simulink model "AutomatedParkingValet"  (R2022b)
settings: Solver=ode23tb  StartTime=0.0  StopTime=inf  FixedStep=1e-3  MaxStep=1e-2  MinStep=1e-3  RelTol=5e-3
PreLoadFcn:
  | costmap = helperSLCreateCostmap();
  | routeData= load('routePlanSL.mat');
  | routePlan= routeData.routePlan;
  | startPose = routePlan.StartPose(1, :);
  | centerToFront = 1.4;
  | centerToRear = 1.4;
  | helperSLCreateUtilityBus;
StopFcn:
  | clear helperSLVisualizePath
libraries: drivinglib x2, simulink x2, simulink_extras x2, autolibshared x1
CloseFcn:
  | clear plannerConfigBus ...
  | speedConfigBus ...
  | startPose ...
  | costmap ...
  | routeData ...
  | routePlan ...
  | centerToFront ...
  | centerToRear;
settings Model: Creator=The MathWorks, Inc.  LastModifiedBy=The MathWorks, Inc.
settings SolverCC: ZeroCrossAlgorithm=Adaptive  AlgebraicLoopSolver=TrustRegion  DecoupledContinuousIntegration=on  MinimalZcImpactIntegration=on
settings DataIOCC: SaveOutput=off  SignalLogging=off  DSMLogging=off  SaveTime=off  ReturnWorkspaceOutputs=off
settings DebuggingCC: UnconnectedInputMsg=warning  UnconnectedOutputMsg=warning  UnconnectedLineMsg=warning  PregeneratedLibrarySubsystemCodeDiagnostic=none  SFMachineParentedDataDiag=warning  ArithmeticOperatorsInVariantConditions=warning
settings ModelReferenceCC: EnableRefExpFcnMdlSchedulingChecks=on
settings SFSimCC: SimUseLocalCustomCode=off
settings RTWCC: RTWUseLocalCustomCode=off

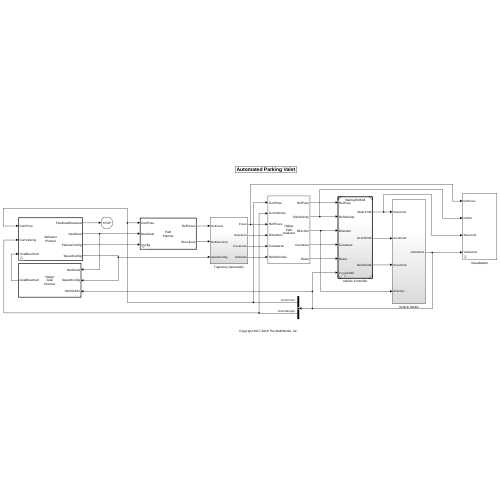
[thumbnail: Simulink's stored preview of the top-level diagram]
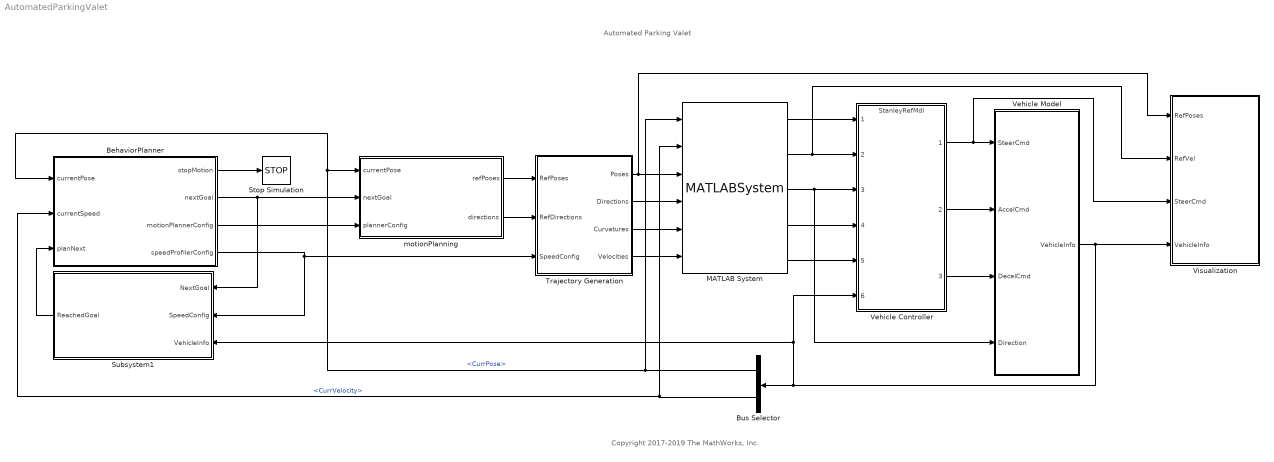
== system AutomatedParkingValet ==
  note: Copyright 2017-2019 The MathWorks, Inc.
  note: Automated Parking Valet
  BehaviorPlanner : MATLAB Function  TreatAsAtomicUnit=on  mask{Costmap=costmap, RoutePlan=routePlan, StartSpeed=0}
      mask prompts: Costmap "Vehicle costmap:"; RoutePlan "Route plan:"; StartSpeed "Initial vehicle speed  [m/s]:"
      mask init:
      | validateattributes(Costmap, {'vehicleCostmap'}, {'scalar'});
      | validateattributes(RoutePlan, {'table'}, {'ncols', 3});
      | validateattributes(StartSpeed, {'double'}, {'scalar','nonnegative'})
      | 
      | routePlanStruct   = table2struct(RoutePlan);
      | startPose         = routePlanStruct(1).StartPose;
      | 
      | varagout          = helperSLCreateUtilityStruct(Costmap);
      | vehicleDimsStruct = varagout{1};
      | costmapStruct     = varagout{2};
  Bus Selector : BusSelector  OutputSignals=CurrPose,CurrVelocity
  MATLAB System : MATLABSystem  System=HelperPathAnalyzer  Wheelbase=2.8  HasResetOutput=on  SimulateUsing=Interpreted execution
      mask Type: HelperPathAnalyzer
      mask Display:
      | disp(['Helper' char(10) 'Path' char(10) 'Analyzer']);
      | port_label('input',1,'CurrPose');
      | port_label('input',2,'CurrVelocity');
      | port_label('input',3,'RefPoses');
      | port_label('input',4,'Directions');
      | port_label('input',5,'Curvatures');
      | port_label('input',6,'RefVelocities');
      | port_label('output',1,'RefPose');
      | port_label('output',2,'RefVelocity');
      | port_label('output',3,'Direction');
      | port_label('output',4,'Curvature');
      | port_label('output',5,'Reset');
  Stop Simulation : Stop
  Subsystem1 : Subsystem  TreatAsAtomicUnit=on  SystemSampleTime=0.1
      settings: MinAlgLoopOccurrences=on
      mask Display:
      | disp(['Helper' char(10) 'Goal' char(10) 'Checker']);
      | port_label('input',1,'NextGoal');
      | port_label('input',2,'SpeedConfig');
      | port_label('input',3,'VehicleInfo');
      | port_label('output',1,'GoalReached');
  Trajectory Generation : Subsystem
  Vehicle Controller : ModelReference  ModelNameDialog=StanleyRefMdl  SimulationMode=Normal  ModelReferenceVersion=1.948
  Vehicle Model : Subsystem
  Visualization : Subsystem  mask{Costmap=costmap}
      mask prompts: Costmap "Vehicle costmap:"
      mask init:
      | validateattributes(Costmap, {'vehicleCostmap'}, {'scalar'});
      | 
      | varagout          = helperSLCreateUtilityStruct(Costmap);
      | vehicleDimsStruct = varagout{1};
      | costmapStruct     = varagout{2};
      mask DialogControl DescTextVar Prompt: Visualize simulation results.
  motionPlanning : MATLAB Function  TreatAsAtomicUnit=on  mask{Costmap=costmap}
      mask prompts: Costmap "Vehicle costmap:"
      mask init:
      | validateattributes(Costmap, {'vehicleCostmap'}, {'scalar'});
      | 
      | varagout          = helperSLCreateUtilityStruct(Costmap);
      | vehicleDimsStruct = varagout{1};
      | costmapStruct     = varagout{2};
  wires:
  BehaviorPlanner/2(nextGoal) -> Subsystem1/1(NextGoal), motionPlanning/2(nextGoal)
  BehaviorPlanner/3(motionPlannerConfig) -> motionPlanning/3(plannerConfig)
  BehaviorPlanner/1(stopMotion) -> Stop Simulation/1
  BehaviorPlanner/4(speedProfilerConfig) -> Subsystem1/2(SpeedConfig), Trajectory Generation/3(SpeedConfig)
  Subsystem1/1(ReachedGoal) -> BehaviorPlanner/3(planNext)
  MATLAB System/3 -> Vehicle Controller/3, Vehicle Model/4(Direction)
  MATLAB System/2 -> Vehicle Controller/2, Visualization/2(RefVel)
  MATLAB System/1 -> Vehicle Controller/1
  MATLAB System/4 -> Vehicle Controller/4
  Vehicle Model/1(VehicleInfo) -> Vehicle Controller/6, Subsystem1/3(VehicleInfo), Bus Selector/1, Visualization/4(VehicleInfo)
  Bus Selector/1 -> BehaviorPlanner/1(currentPose), motionPlanning/1(currentPose), MATLAB System/1  "<CurrPose>"
  Bus Selector/2 -> MATLAB System/2, BehaviorPlanner/2(currentSpeed)  "<CurrVelocity>"
  MATLAB System/5 -> Vehicle Controller/5
  Vehicle Controller/3 -> Vehicle Model/3(DecelCmd)
  Vehicle Controller/1 -> Vehicle Model/1(SteerCmd), Visualization/3(SteerCmd)
  Vehicle Controller/2 -> Vehicle Model/2(AccelCmd)
  Trajectory Generation/1(Poses) -> Visualization/1(RefPoses), MATLAB System/3
  motionPlanning/1(refPoses) -> Trajectory Generation/1(RefPoses)
  motionPlanning/2(directions) -> Trajectory Generation/2(RefDirections)
  Trajectory Generation/2(Directions) -> MATLAB System/4
  Trajectory Generation/3(Curvatures) -> MATLAB System/5
  Trajectory Generation/4(Velocities) -> MATLAB System/6

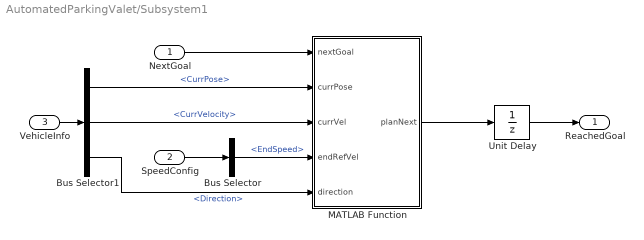
== system AutomatedParkingValet/Subsystem1 ==
  NextGoal : Inport
  SpeedConfig : Inport  Port=2
  VehicleInfo : Inport  Port=3
  Bus Selector : BusSelector  OutputSignals=EndSpeed
  Bus Selector1 : BusSelector  OutputSignals=CurrPose,CurrVelocity,Direction
  MATLAB Function : MATLAB Function  TreatAsAtomicUnit=on
  Unit Delay : UnitDelay  SampleTime=-1  HasFrameUpgradeWarning=on
  ReachedGoal : Outport  VectorParamsAs1DForOutWhenUnconnected=off
  wires:
  Bus Selector1/1 -> MATLAB Function/2(currPose)  "<CurrPose>"
  VehicleInfo/1 -> Bus Selector1/1
  Bus Selector1/3 -> MATLAB Function/5(direction)  "<Direction>"
  Bus Selector/1 -> MATLAB Function/4(endRefVel)  "<EndSpeed>"
  Unit Delay/1 -> ReachedGoal/1
  SpeedConfig/1 -> Bus Selector/1
  MATLAB Function/1(planNext) -> Unit Delay/1
  Bus Selector1/2 -> MATLAB Function/3(currVel)  "<CurrVelocity>"
  NextGoal/1 -> MATLAB Function/1(nextGoal)

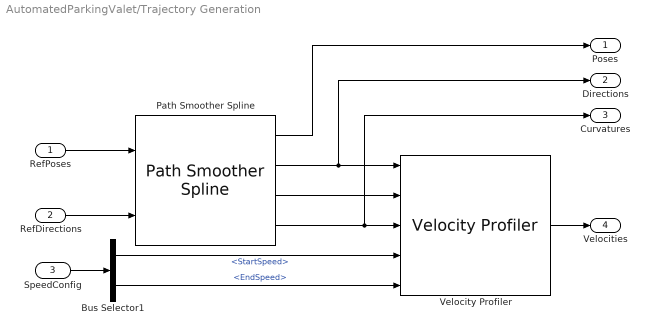
== system AutomatedParkingValet/Trajectory Generation ==
  RefPoses : Inport
  RefDirections : Inport  Port=2
  SpeedConfig : Inport  Port=3
  Bus Selector1 : BusSelector  OutputSignals=StartSpeed,EndSpeed
  Path Smoother Spline : drivinglib/Path Smoother Spline  NumSmoothPoses=500  MinSeparation=1e-3  SampleTime=-1  ShowOptionalOutports=on  SimulateUsing=Interpreted execution
  Velocity Profiler : drivinglib/Velocity Profiler  MaxLongitudinalAccel=2  MaxLongitudinalDecel=4  MaxSpeed=10  MaxLongitudinalJerk=1  MaxLateralAccel=2  ShowOptionalOutport=off  SampleTime=-1  SimulateUsing=Interpreted execution
  Poses : Outport  VectorParamsAs1DForOutWhenUnconnected=off
  Directions : Outport  Port=2  VectorParamsAs1DForOutWhenUnconnected=off
  Curvatures : Outport  Port=3  VectorParamsAs1DForOutWhenUnconnected=off
  Velocities : Outport  Port=4  VectorParamsAs1DForOutWhenUnconnected=off
  wires:
  Velocity Profiler/1 -> Velocities/1
  Path Smoother Spline/2 -> Directions/1, Velocity Profiler/1
  Path Smoother Spline/4 -> Curvatures/1, Velocity Profiler/3
  Bus Selector1/2 -> Velocity Profiler/5  "<EndSpeed>"
  RefPoses/1 -> Path Smoother Spline/1
  SpeedConfig/1 -> Bus Selector1/1
  Bus Selector1/1 -> Velocity Profiler/4  "<StartSpeed>"
  Path Smoother Spline/3 -> Velocity Profiler/2
  RefDirections/1 -> Path Smoother Spline/2
  Path Smoother Spline/1 -> Poses/1

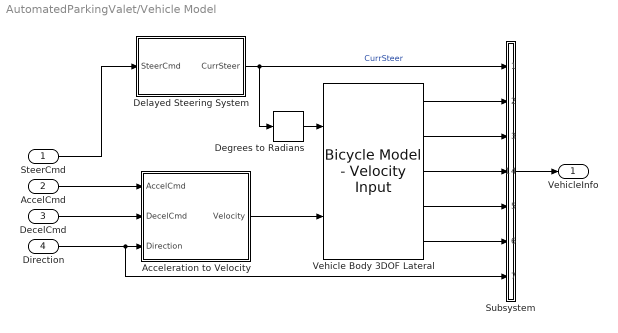
== system AutomatedParkingValet/Vehicle Model ==
  SteerCmd : Inport
  AccelCmd : Inport  Port=2
  DecelCmd : Inport  Port=3
  Direction : Inport  Port=4
  Acceleration to Velocity : Subsystem  TreatAsAtomicUnit=on
  Degrees to Radians : simulink_extras/Transformations/Degrees to Radians
  Delayed Steering System : Subsystem
  Subsystem : Subsystem
  Vehicle Body 3DOF Lateral : autolibshared/Bicycle Model - Velocity Input  trackMode=Single (bicycle)  inputMode=External longitudinal forces  frontSteerMode=on  rearSteerMode=off  windMode=off  muMode=off  extFMode=off  extMMode=off  aMode=3  NF=2  NR=2  m=1575  a=1.2  b=1.6  h=0.35  X_o=startPose(1)+cosd(startPose(3))*1.6  xdot_o=0  CalphaMode=off  sigmaMode=on  w=[1.4,1.4]  Cy_f=19e3  Cy_r=20e3  sigma_f=.1  sigma_r=.1  alpha_f_brk=[-.1 .1]  Cy_f_data=[-9e3 9e3]  alpha_r_brk=[-.1 .1]  Cy_r_data=[-9e3 9e3]  Y_o=startPose(2) +sind(startPose(3))*1.6  ydot_o=0  Izz=4000  psi_o=deg2rad(startPose(3))  r_o=0  Af=2  Cd=.3  Cl=.1  Cpm=.1  beta_w=[0:0.01:0.3]  Cs=[0:0.03:0.9]  Cym=[0:0.01:0.3]  Pabs=101325  Tair=273  g=9.81  mu=1  xdot_tol=0.01  Fznom=5000  Fxtire_sat=1e6  Fytire_sat=1e6  longOff=0  latOff=0  vertOff=0
  VehicleInfo : Outport  VectorParamsAs1DForOutWhenUnconnected=off
  wires:
  Acceleration to Velocity/1(Velocity) -> Vehicle Body 3DOF Lateral/2
  Direction/1 -> Subsystem/7(<Direction>), Acceleration to Velocity/3(Direction)
  Degrees to Radians/1 -> Vehicle Body 3DOF Lateral/1
  Delayed Steering System/1(CurrSteer) -> Degrees to Radians/1, Subsystem/1(CurrSteer)  "CurrSteer"
  DecelCmd/1 -> Acceleration to Velocity/2(DecelCmd)
  AccelCmd/1 -> Acceleration to Velocity/1(AccelCmd)
  SteerCmd/1 -> Delayed Steering System/1(SteerCmd)
  Subsystem/1(VehicleInfo) -> VehicleInfo/1
  Vehicle Body 3DOF Lateral/1 -> Subsystem/2(Info)
  Vehicle Body 3DOF Lateral/2 -> Subsystem/3(In3)
  Vehicle Body 3DOF Lateral/3 -> Subsystem/4(In4)
  Vehicle Body 3DOF Lateral/4 -> Subsystem/5(In5)
  Vehicle Body 3DOF Lateral/5 -> Subsystem/6(In6)

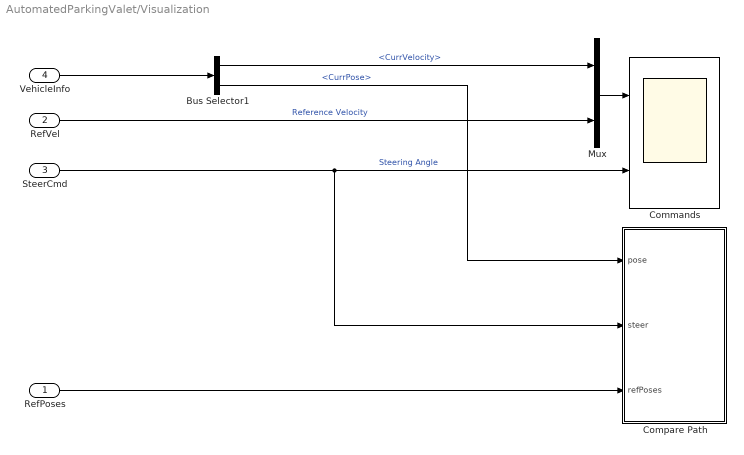
== system AutomatedParkingValet/Visualization ==
  RefPoses : Inport
  RefVel : Inport  Port=2
  SteerCmd : Inport  Port=3
  VehicleInfo : Inport  Port=4
  Bus Selector1 : BusSelector  OutputSignals=CurrVelocity,CurrPose
  Commands : Scope  NumInputPorts=2
  Compare Path : MATLAB Function  TreatAsAtomicUnit=on
  Mux : Mux  Inputs=2
  wires:
  RefPoses/1 -> Compare Path/3(refPoses)
  Bus Selector1/1 -> Mux/1  "<CurrVelocity>"
  Bus Selector1/2 -> Compare Path/1(pose)  "<CurrPose>"
  RefVel/1 -> Mux/2  "Reference Velocity"
  Mux/1 -> Commands/1
  SteerCmd/1 -> Compare Path/2(steer), Commands/2  "Steering Angle"
  VehicleInfo/1 -> Bus Selector1/1

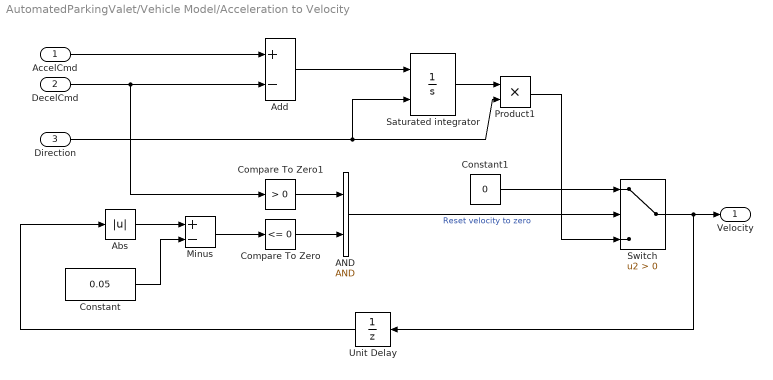
== system AutomatedParkingValet/Vehicle Model/Acceleration to Velocity ==
  AccelCmd : Inport  PortDimensions=[1 1]
  DecelCmd : Inport  Port=2  PortDimensions=[1 1]
  Direction : Inport  Port=3
  AND : Logic  IconShape=distinctive  AllPortsSameDT=off  OutDataTypeStr=boolean
  Abs : Abs  SaturateOnIntegerOverflow=off
  Add : Sum  Inputs=+-
  Compare To Zero : simulink/Logic and Bit Operations/Compare To Zero  relop=<=  OutDataTypeStr=boolean
  Compare To Zero1 : simulink/Logic and Bit Operations/Compare To Zero  relop=>  OutDataTypeStr=boolean
  Constant : Constant  Value=0.05
  Constant1 : Constant  Value=0
  Minus : Sum  Inputs=+-
  Product1 : Product
  Saturated integrator : Integrator  ExternalReset=either  LimitOutput=on  LowerSaturationLimit=0  AbsoluteTolerance=1e-3  ZeroCross=off
  Switch : Switch  Criteria=u2 > Threshold  SaturateOnIntegerOverflow=off  InputSameDT=off
  Unit Delay : UnitDelay  SampleTime=-1  HasFrameUpgradeWarning=on
  Velocity : Outport  VectorParamsAs1DForOutWhenUnconnected=off
  wires:
  Direction/1 -> Product1/2, Saturated integrator/2
  AccelCmd/1 -> Add/1
  Add/1 -> Saturated integrator/1
  DecelCmd/1 -> Compare To Zero1/1, Add/2
  Unit Delay/1 -> Abs/1
  Abs/1 -> Minus/1
  Constant/1 -> Minus/2
  Minus/1 -> Compare To Zero/1
  Compare To Zero/1 -> AND/2
  Compare To Zero1/1 -> AND/1
  AND/1 -> Switch/2  "Reset velocity to zero"
  Switch/1 -> Unit Delay/1, Velocity/1
  Constant1/1 -> Switch/1
  Saturated integrator/1 -> Product1/1
  Product1/1 -> Switch/3

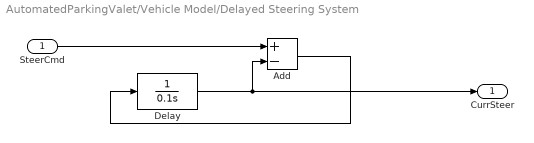
== system AutomatedParkingValet/Vehicle Model/Delayed Steering System ==
  SteerCmd : Inport
  Add : Sum  Inputs=+-
  Delay : TransferFcn  Denominator=[0.1 0]
  CurrSteer : Outport  VectorParamsAs1DForOutWhenUnconnected=off
  wires:
  Add/1 -> Delay/1
  SteerCmd/1 -> Add/1
  Delay/1 -> CurrSteer/1, Add/2

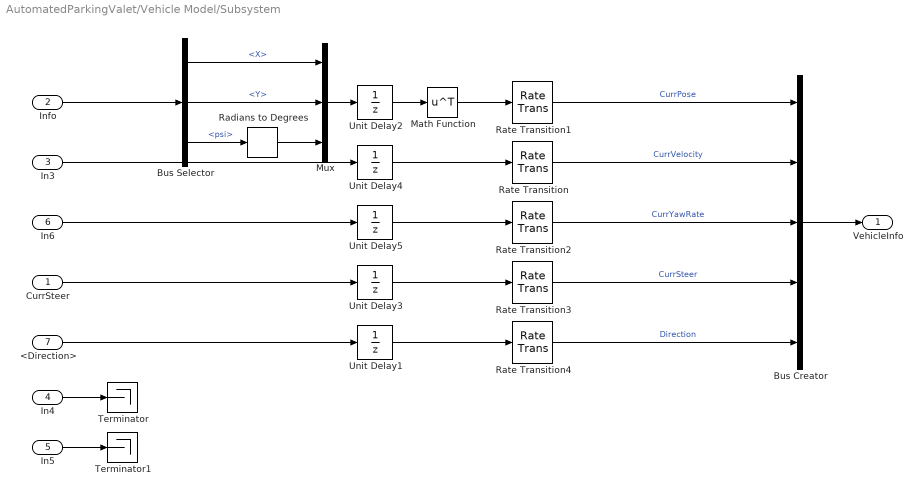
== system AutomatedParkingValet/Vehicle Model/Subsystem ==
  CurrSteer : Inport
  Info : Inport  Port=2
  In3 : Inport  Port=3
  In4 : Inport  Port=4
  In5 : Inport  Port=5
  In6 : Inport  Port=6
  <Direction> : Inport  Port=7
  Bus Creator : BusCreator  Inputs=5  OutDataTypeStr=Bus: vehicleInfoBus  NonVirtualBus=on
  Bus Selector : BusSelector  OutputSignals=InertFrm.RearAxl.Disp.X,InertFrm.RearAxl.Disp.Y,InertFrm.Cg.Ang.psi
  Math Function : Math  Operator=transpose  SignedPower=on
  Mux : Mux  Inputs=3
  Radians to Degrees : simulink_extras/Transformations/Radians to Degrees
  Rate Transition : RateTransition  OutPortSampleTime=0.05
  Rate Transition1 : RateTransition  InitialCondition=startPose  OutPortSampleTime=0.05
  Rate Transition2 : RateTransition  OutPortSampleTime=0.05
  Rate Transition3 : RateTransition  OutPortSampleTime=0.05
  Rate Transition4 : RateTransition  InitialCondition=1  OutPortSampleTime=0.05
  Terminator : Terminator
  Terminator1 : Terminator
  Unit Delay1 : UnitDelay  InitialCondition=1  SampleTime=-1  HasFrameUpgradeWarning=on
  Unit Delay2 : UnitDelay  InitialCondition=startPose  SampleTime=-1  HasFrameUpgradeWarning=on
  Unit Delay3 : UnitDelay  SampleTime=-1  HasFrameUpgradeWarning=on
  Unit Delay4 : UnitDelay  SampleTime=-1  HasFrameUpgradeWarning=on
  Unit Delay5 : UnitDelay  SampleTime=-1  HasFrameUpgradeWarning=on
  VehicleInfo : Outport  VectorParamsAs1DForOutWhenUnconnected=off
  wires:
  Unit Delay1/1 -> Rate Transition4/1
  CurrSteer/1 -> Unit Delay3/1
  Unit Delay5/1 -> Rate Transition2/1
  <Direction>/1 -> Unit Delay1/1
  Unit Delay4/1 -> Rate Transition/1
  Math Function/1 -> Rate Transition1/1
  Rate Transition/1 -> Bus Creator/2  "CurrVelocity"
  Unit Delay3/1 -> Rate Transition3/1
  Rate Transition3/1 -> Bus Creator/4  "CurrSteer"
  Rate Transition1/1 -> Bus Creator/1  "CurrPose"
  Rate Transition2/1 -> Bus Creator/3  "CurrYawRate"
  Rate Transition4/1 -> Bus Creator/5  "Direction"
  In5/1 -> Terminator1/1
  Unit Delay2/1 -> Math Function/1
  Info/1 -> Bus Selector/1
  Radians to Degrees/1 -> Mux/3
  Bus Selector/2 -> Mux/2  "<Y>"
  Bus Selector/1 -> Mux/1  "<X>"
  Mux/1 -> Unit Delay2/1
  In3/1 -> Unit Delay4/1
  In4/1 -> Terminator/1
  In6/1 -> Unit Delay5/1
  Bus Selector/3 -> Radians to Degrees/1  "<psi>"
  Bus Creator/1 -> VehicleInfo/1

== matlab function AutomatedParkingValet/motionPlanning ==
  settings: updateMethod=DISCRETE  sampleTime=0.1
  data: refPoses output size=[100 3]; currentPose input size=[1 3]; nextGoal input size=[1 3]; plannerConfig input Bus: plannerConfigBus; costmapStruct parameter; vehicleDimsStruct parameter; directions output size=[100 1]
function [refPoses, directions] = motionPlanning(currentPose, nextGoal, ...
    plannerConfig, costmapStruct, vehicleDimsStruct)

%motionPlanning plan a feasible path using pathPlannerRRT.

%#codegen

persistent nextGoalPose posesInternal directionsInternal

% Initialize persistent variables
if isempty(nextGoalPose)
    nextGoalPose = [0 0 0];
end

if isempty(posesInternal)
    posesInternal = [0 0 0];
end

if isempty(directionsInternal)
    directionsInternal = 1;
end

% Create vehicleDimensions object
vehicleDims = vehicleDimensions( ...
    vehicleDimsStruct.Length, ...
    vehicleDimsStruct.Width, ...
    vehicleDimsStruct.Height, ...
    'Wheelbase',          vehicleDimsStruct.Wheelbase, ...
    'RearOverhang',       vehicleDimsStruct.RearOverhang, ...
    'WorldUnits',         char(vehicleDimsStruct.WorldUnits));

ccConfig = inflationCollisionChecker(vehicleDims, 4);

% Initialize vehicleCostmap object
costmap = vehicleCostmap(costmapStruct.Costs, ...
    'FreeThreshold',      costmapStruct.FreeThreshold, ...
    'OccupiedThreshold',  costmapStruct.OccupiedThreshold, ...
    'MapLocation',        costmapStruct.MapExtent([1, 3]), ...
    'CellSize',           costmapStruct.CellSize, ...
    'CollisionChecker',   ccConfig);

% Create pathPlannerRRT object
motionPlanner = pathPlannerRRT(costmap, ...
    'ConnectionDistance', plannerConfig.ConnectionDistance, ...
    'MinIterations',      plannerConfig.MinIterations, ...
    'GoalTolerance',      plannerConfig.GoalTolerance, ...
    'MinTurningRadius',   plannerConfig.MinTurningRadius);

% Only plan the path if there is a new goal
if ~isequal(nextGoalPose, nextGoal)
    nextGoalPose  = nextGoal;
    vehiclePose   = currentPose;
    refPath       = plan(motionPlanner, vehiclePose, nextGoalPose);
    [refPoses, directions] = interpolate(refPath);
    posesInternal          = refPoses;
    directionsInternal     = directions;
else
    refPoses   = posesInternal;
    directions = directionsInternal;
end

if isempty(refPoses)
    error('No feasible path can be found.')
end

end

== matlab function AutomatedParkingValet/Subsystem1/MATLAB Function ==
  data: nextGoal input size=[1 3]; planNext output size=[1 1]; currPose input size=[1 3]; currVel input size=[1 1]; endRefVel input size=[1 1]; direction input
function planNext = goalChecker(nextGoal, currPose, currVel, endRefVel, direction)

planNext = helperGoalChecker(nextGoal, currPose, currVel, endRefVel, direction);

== matlab function AutomatedParkingValet/Visualization/Compare Path ==
  settings: updateMethod=DISCRETE  sampleTime=0.1
  data: pose input size=[1 3]; steer input; refPoses input; costmapStruct parameter; vehicleDimsStruct parameter
function visualizePath(pose, steer, refPoses, costmapStruct, vehicleDimsStruct)

%visualizePath Display simulation results.

coder.extrinsic('helperSLVisualizePath');

helperSLVisualizePath(pose, steer, refPoses, costmapStruct, vehicleDimsStruct)

== matlab function AutomatedParkingValet/BehaviorPlanner ==
  settings: updateMethod=DISCRETE  sampleTime=0.1
  data: stopMotion output; nextGoal output double size=[1 3]; motionPlannerConfig output Bus: plannerConfigBus; speedProfilerConfig output Bus: speedConfigBus; routePlanStruct parameter; currentPose input size=[1 3]; currentSpeed input size=[1 1]; planNext input size=[1 1]; startPose parameter size=[1 3]; StartSpeed parameter
function [stopMotion, nextGoal, motionPlannerConfig, speedProfilerConfig] = ...
    behaviorPlanning(routePlanStruct, currentPose, currentSpeed, planNext, ...
    startPose, StartSpeed)

%behaviorPlanning generate navigation tasks and configurations for the 
%   Motion Planner block and the Trajectory Generator block.

nextGoal     = coder.nullcopy(zeros(1, 3)); %#ok<*NASGU>
stopMotion   = coder.nullcopy(logical(0));  %#ok<*LOGL>

persistent behavioralPlanner
persistent nextGoalPose plannerConfig speedConfig
persistent pose speed

if isempty(behavioralPlanner)
    
    % Initialize pose and speed
    pose  = startPose;
    speed = StartSpeed;
    
    % Initialize planner
    steerLimit = 30;
    behavioralPlanner = HelperBehavioralPlanner(routePlanStruct, steerLimit);
    [nextGoalPose, plannerConfig, speedConfig] = requestManeuver( ...
        behavioralPlanner, pose, speed);
end

pose  = currentPose;
speed = currentSpeed;

disTol = 1;
% Plan a new path when reaching the goal
if planNext && ~reachedDestination(behavioralPlanner)
    [nextGoalPose, plannerConfig, speedConfig] = requestManeuver( ...
        behavioralPlanner, pose, speed);
end

% Stop motion when reaching the destination
stopMotion = planNext && reachedDestination(behavioralPlanner) && ...
    norm(pose(1:2) - nextGoalPose(1:2)) < disTol;
    
nextGoal            = nextGoalPose;
motionPlannerConfig.ConnectionDistance = plannerConfig.ConnectionDistance;
motionPlannerConfig.MinIterations = plannerConfig.MinIterations;
motionPlannerConfig.GoalTolerance = plannerConfig.GoalTolerance;
motionPlannerConfig.MinTurningRadius = plannerConfig.MinTurningRadius;
speedProfilerConfig = speedConfig;

end
